simulink model "HvCoorn"  (R2022b)
settings: configuration reference "Icar05FusaMdlCfg" (kept outside this file)
undefined symbols (not defined in the file): BMSActSt_ACChrg, BMSActSt_DCChrg, BMSActSt_disconnect, BMSActSt_offline, BMSActSt_online, BMSActSt_undefined, BMSMainNegRlySt_Clsd_SC, BMSMainNegRlySt_Open_SC, BMSMainNegRlySt_StuckInClsd_SC, BMSMainNegRlySt_StuckInOpen_SC, BMSMainPosRlySt_Clsd_SC, BMSMainPosRlySt_Open_SC, BMSMainPosRlySt_StuckInClsd_SC, BMSPrecRlySt_StuckInOpen_SC, BMSReqSt_ACChrg, BMSReqSt_DCChrg, BMSReqSt_emergencyOffline, BMSReqSt_offline, BMSReqSt_online, Chrg_stCycleBookMod_SC, Chrg_stSingleBookMod_SC, CmpgMod_stInactv_SC, DCDCActSt_buck, DCDCActSt_connected, DCDCActSt_disconnected, DCDCReqSt_buck, DCDCReqSt_standby, EngStrtStop_RefuModDft_SC, EPBActSt_Appld_SC, GearLvr_stDrvGearD_SC, GearLvr_stDrvGearN_SC, GearLvr_stDrvGearP_SC, GearLvr_stDrvGearR_SC, hpp_bACChargeLinkIni_C, hpp_bACChargeLinkOKIni_C, hpp_bAcChgEnaIni_C, hpp_bAcChgPauseIni_C, hpp_bAcLinkTempErrIni_C, hpp_bBattWarmReqIni_C, hpp_bHvilHwErrIni_C, hpp_bHvilStOkIni_C, hpp_bHvRelayClsActIni_C, hpp_bHvRelayOpnActIni_C, hpp_bHvRelayStuckIni_C, hpp_bParked4ChDchgIni_C, hpp_bRemLvBatMntnReqIni_C, hpp_bStartUpReqIni_C, hpp_stHvilCanIni_C, hpp_stWarmTimeCfgRespIni_C, HvCoorn_bAuthEnaSwt_C, HvCoorn_bAuthFailSpdLimOvrd_C, HvCoorn_bAuthFailSpdLimOvrdVal_C, HvCoorn_bAuthStrt_C, HvCoorn_bBMSUnexpdDcnctFailEna_C, HvCoorn_bBuck2RdyBypDCDCEna_C, HvCoorn_bDCChrgFctCfg_C, HvCoorn_bDcChrgWkupEnaChrgLink_C, HvCoorn_bDCDcnct4ACEna_C, HvCoorn_bDCNotBuck2ShtdwnEna_C, HvCoorn_bDrvrLevNotRdyEna_C ... (+295)
libraries: ITKLib x213, simulink x61
(part 11 of 12)

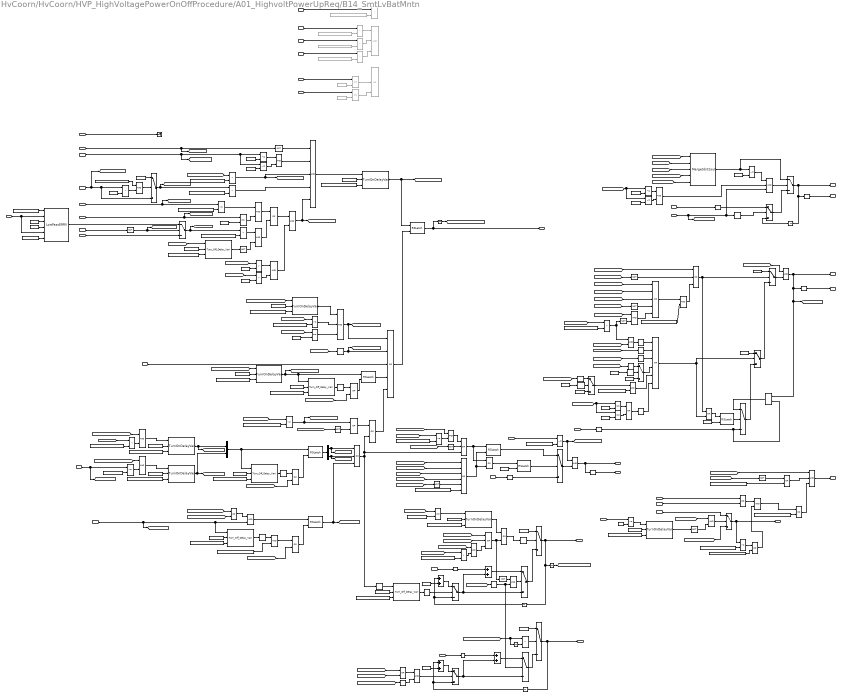
== system HvCoorn/HvCoorn/HVP_HighVoltagePowerOnOffProcedure/A01_HighvoltPowerUpReq/B14_SmtLvBatMntn ==
  icebs_pctLvBatSoh : Inport
  icbms_pctHVBatSOCDisp : Inport  Port=2
  icbms_tMaxBat : Inport  Port=3
  icbms_tMinBat : Inport  Port=4
  icebs_tLvBat : Inport  Port=5
  icebs_pctLvBatSoc : Inport  Port=6
  icebs_stSocPrcsn : Inport  Port=7
  icebs_uLvBat : Inport  Port=8
  idi_bKeyOn : Inport  Port=9
  ved_bInhbHvOn : Inport  Port=10
  icdc_stMode : Inport  Port=11
  icicm_bOTAOn : Inport  Port=12
  icicm_stHVReq : Inport  Port=13
  icicm_stOTAPwrMngtReq : Inport  Port=14
  HvCoorn_ctSmtBatMntnFailEER : Inport  Port=15
  iud_bEEIniFnsd : Inport  Port=16
  HvCoorn_stHVPOld : Inport  Port=17
  HvCoorn_ctSmtBatMntnSucsEER : Inport  Port=18
  ipf_bBD1CAN0x41CVld : Inport  Port=19
  idi_uPwrSply : Inport  Port=20
  ipf_bLIN9EBS0x34NodLostErr : Inport  Port=21
  HvCoorn_bSocWkupEER : Inport  Port=22
  HvCoorn_bTimerWkupReqEER : Inport  Port=23
  HvCoorn_stRemLvBatMntnFailRsnEER : Inport  Port=24
  idi_bEBSLinWkup : Inport  Port=25
  idi_bTimerWkup : Inport  Port=26
  HvCoorn_pctHVBatSocEER : Inport  Port=27
  idi_noBMSSocCounter : Inport  Port=28
  VehCfg_stLvBattTyp : Inport  Port=29
  AND : Logic  Inputs=5  OutDataTypeStr=boolean
  AND{1,6..7,9..10,12,17..20,22,24,26,29..30,32,36..40} (21 alike) : Logic  OutDataTypeStr=boolean
  AND{3,11,14,25,33..34} (6 alike) : Logic  Operator=OR  OutDataTypeStr=boolean
  AND13 : Logic  Operator=OR  Inputs=3  OutDataTypeStr=boolean
  AND15 : Logic  Operator=NOT  Inputs=3  OutDataTypeStr=boolean
  AND16 : Logic  Operator=NOT  Inputs=3  OutDataTypeStr=boolean
  AND2 : Logic  Commented=on  Inputs=3  OutDataTypeStr=boolean
  AND21 : Logic  Operator=OR  Inputs=6  OutDataTypeStr=boolean
  AND23 : Logic  Inputs=3  OutDataTypeStr=boolean
  AND27 : Logic  Operator=OR  Inputs=3  OutDataTypeStr=boolean
  AND28 : Logic  Operator=OR  Inputs=3  OutDataTypeStr=boolean
  AND31 : Logic  Operator=OR  Inputs=5  OutDataTypeStr=boolean
  AND35 : Logic  Inputs=3  OutDataTypeStr=boolean
  AND4 : Logic  Operator=OR  Inputs=5  OutDataTypeStr=boolean
  AND5 : Logic  Inputs=3  OutDataTypeStr=boolean
  AND8 : Logic  Commented=on  Operator=OR  Inputs=3  OutDataTypeStr=boolean
  Add{,1..3} (4 alike) : Sum  InputSameDT=on  SaturateOnIntegerOverflow=on
  Constant84 : Constant  Description=[1]  Value=LvBattTyp_stLiBatt_SC
      settings: AttributesFormatString=%<Description>
  CrCtl_tiFltVeh_C : Constant  Description=[0.02]  Value=HvCoorn_tiFiltLvVolt_C  SampleTime=-1
      settings: AttributesFormatString=%<Description>  CopyFcn=if exist('tl_reset_reviewflag','file')==2,tl_reset_reviewflag(gcbh);end  DeleteFcn=if exist('delete_tlblock','file')==2,delete_tlblock(gcbh);end  NameChangeFcn=if exist('rename_tlblock','file')==2,rename_tlblock(gcbh);end  OpenFcn=if exist('tl_open_blockdlg','file')==2,tl_open_blockdlg(gcbh);else,open_system(gcbh,'parameter');end
  Delay : Delay  DelayLength=1  InitialConditionSource=Input port
      settings: InputPortMap=u0,p4
  Delay1 : Delay  DelayLength=10  InitialCondition=0
  Delay2 : Delay  DelayLength=500  InitialCondition=0
  Demux : Demux  Outputs=2
  EdgeFalling{,1..3,5..6} (6 alike) : ITKLib/Memory/EdgeFalling  Tag=initial value = 0
      settings: SourceProductName=ITKC_Lib
  EdgeRising{,1..6,8,11..12} (10 alike) : ITKLib/Memory/EdgeRising  Tag=initial value = 0
      settings: SourceProductName=ITKC_Lib
  Equal : RelationalOperator  Commented=on  Operator===  OutDataTypeStr=boolean  RndMeth=Simplest  InputSameDT=off
  Equal1 : RelationalOperator  Commented=on  Operator===  OutDataTypeStr=boolean  RndMeth=Simplest  InputSameDT=off
  Equal2 : RelationalOperator  Operator=<  OutDataTypeStr=boolean
  Equal3 : RelationalOperator  Operator=~=  OutDataTypeStr=boolean
  Equal4 : RelationalOperator  Operator=~=  OutDataTypeStr=boolean
  Equal5 : RelationalOperator  OutDataTypeStr=boolean
  Equal7 : RelationalOperator  Operator=~=  OutDataTypeStr=boolean
  FALSE{1..4,6} (5 alike) : Constant  Description=FALSE  Value=0  OutDataTypeStr=boolean  SampleTime=-1
      settings: AttributesFormatString=%<Description>
  FALSE5 : Constant  Description=FALSE  Value=0  OutDataTypeStr=boolean
      settings: AttributesFormatString=%<Description>
  Greater : RelationalOperator  Commented=on  Operator=>  OutDataTypeStr=boolean
  Greater1 : RelationalOperator  Operator=<  OutDataTypeStr=boolean
  Greater{7,10..11,21} (4 alike) : RelationalOperator  Operator===  OutDataTypeStr=boolean
  Greater12 : RelationalOperator  Operator=<  OutDataTypeStr=boolean
  Greater{2,13..14,17..19} (6 alike) : RelationalOperator  Operator=>  OutDataTypeStr=boolean
  Greater{15..16,20,22} (4 alike) : RelationalOperator  Operator=~=  OutDataTypeStr=boolean
  Greater23 : RelationalOperator  Operator=<=  OutDataTypeStr=boolean
  Greater26 : RelationalOperator  Operator=<=  OutDataTypeStr=boolean
  Greater3 : RelationalOperator  Commented=on  Operator=>  OutDataTypeStr=boolean
  Greater4 : RelationalOperator  Commented=on  Operator=<  OutDataTypeStr=boolean
  Greater5 : RelationalOperator  Commented=on  Operator=>  OutDataTypeStr=boolean
  Greater6 : RelationalOperator  Operator=<=  OutDataTypeStr=boolean
  Greater8 : RelationalOperator  Operator=<  OutDataTypeStr=boolean
  Greater9 : RelationalOperator  OutDataTypeStr=boolean
  LowPassERRV1 : ITKLib/Filter/LowPassERRV
      settings: SourceProductName=ITKC_Lib
  Merge5bit2out : ITKLib/BitOperation/Merge5bit2out
      settings: SourceProductName=ITKC_Lib
  Mux : Mux  Inputs=2
  Not{,1..9} (10 alike) : Logic  Operator=NOT  AllPortsSameDT=off  OutDataTypeStr=boolean
  OR : Logic  Operator=OR  Inputs=3  OutDataTypeStr=boolean
  OR1 : Logic  OutDataTypeStr=boolean
  OR{2..5,7..8,10..13} (10 alike) : Logic  Operator=OR  OutDataTypeStr=boolean
  OR6 : Logic  Operator=OR  Inputs=6  OutDataTypeStr=boolean
  OR9 : Logic  OutDataTypeStr=boolean
  RSLatch{,1..6} (7 alike) : ITKLib/Memory/RSLatch
      settings: SourceProductName=ITKC_Lib
  Relational Operator1 : RelationalOperator  Operator===  OutDataTypeStr=boolean  InputSameDT=off
  Relational Operator5 : RelationalOperator  Operator=~=  OutDataTypeStr=boolean  InputSameDT=off
  Signal Copy{,1..7} (8 alike) : SignalConversion  OverrideOpt=off
  Switch{,1..9,11..17} (17 alike) : Switch  Criteria=u2 ~= 0  SaturateOnIntegerOverflow=off  InputSameDT=off
      settings: AttributesFormatString=Criteria : %<Criteria>
  TRUE : Constant  Description=TRUE  OutDataTypeStr=boolean  SampleTime=-1
      settings: AttributesFormatString=%<Description>
  TRUE1 : Constant  Description=TRUE  OutDataTypeStr=boolean  SampleTime=-1
      settings: AttributesFormatString=%<Description>
  TRUE2 : Constant  Description=TRUE  OutDataTypeStr=boolean
      settings: AttributesFormatString=%<Description>
  TRUE3 : Constant  Description=TRUE  OutDataTypeStr=boolean  SampleTime=-1
      settings: AttributesFormatString=%<Description>
  TaskTime_s{1..13} (13 alike) : Constant  Value=TaskTime_10ms
      settings: AttributesFormatString=[0.01]
  Terminator : Terminator
  TurnOnDelayVari{,1..6} (7 alike) : ITKLib/TimeCounter/TurnOnDelayVari
      settings: AttributesFormatString=TurnOnDelay  SourceProductName=ITKC_Lib
  Turn_Off_Delay_Vari{,1..4} (5 alike) : ITKLib/TimeCounter/Turn_Off_Delay_Vari
      settings: AttributesFormatString=TurnOffDelay  SourceProductName=ITKC_Lib
  Unit Delay : UnitDelay  SampleTime=-1  HasFrameUpgradeWarning=on
      settings: AttributesFormatString=<initial=%<x0>>
  Unit Delay1 : UnitDelay  SampleTime=-1  HasFrameUpgradeWarning=on
      settings: AttributesFormatString=<initial=%<x0>>
  Unit Delay2 : UnitDelay  SampleTime=-1  HasFrameUpgradeWarning=on
      settings: AttributesFormatString=<initial=%<x0>>
  UnitDelay : UnitDelay  SampleTime=-1  HasFrameUpgradeWarning=on
      settings: AttributesFormatString=<Initial=%<x0>>
  UnitDelay1 : UnitDelay  SampleTime=-1  HasFrameUpgradeWarning=on
      settings: AttributesFormatString=<Initial=%<x0>>
  UnitDelay2 : UnitDelay  SampleTime=-1  HasFrameUpgradeWarning=on
      settings: AttributesFormatString=<Initial=%<x0>>
  hpp_tiRemHvBatPrecdngSet_C : Constant  Description=[75]  Commented=on  Value=HvCoorn_pctLvBatSohRemMntnThd_C
      settings: AttributesFormatString=%<Description>
  hpp_tiRemHvBatPrecdngSet_C1 : Constant  Description=[3]  Value=HvCoorn_ctSmtBatMntnFailThd_C
      settings: AttributesFormatString=%<Description>
  hpp_tiRemHvBatPrecdngSet_C10 : Constant  Description=[70]  Value=HvCoorn_pctHvBatSocMntnFailClr_C
      settings: AttributesFormatString=%<Description>
  hpp_tiRemHvBatPrecdngSet_C11 : Constant  Description=[5400]  Value=HvCoorn_tiRemMntnActvOverThd_C
      settings: AttributesFormatString=%<Description>
  hpp_tiRemHvBatPrecdngSet_C12 : Constant  Description=[15]  Value=HvCoorn_tiRemMntnDcdcNoBuckEx_C
      settings: AttributesFormatString=%<Description>
  hpp_tiRemHvBatPrecdngSet_C13 : Constant  Description=[13]  Value=HvCoorn_uLvBatRemMntnExThd_C
      settings: AttributesFormatString=%<Description>
  hpp_tiRemHvBatPrecdngSet_C14 : Constant  Description=[15]  Value=HvCoorn_tiRemMntnLvVoltExThd_C
      settings: AttributesFormatString=%<Description>
  hpp_tiRemHvBatPrecdngSet_C15 : Constant  Description=[70]  Value=HvCoorn_pctHvBatSocMntnFailClr_C
      settings: AttributesFormatString=%<Description>
  hpp_tiRemHvBatPrecdngSet_C16 : Constant  Description=[70]  Value=HvCoorn_pctHvBatSocMntnFailClr_C
      settings: AttributesFormatString=%<Description>
  hpp_tiRemHvBatPrecdngSet_C17 : Constant  Description=[180]  Value=HvCoorn_tiMntnKeyOffThd_C
      settings: AttributesFormatString=%<Description>
  hpp_tiRemHvBatPrecdngSet_C18 : Constant  Description=[8]  Value=HvCoorn_pctHvBatSocRemMntnExThd_C
      settings: AttributesFormatString=%<Description>
  hpp_tiRemHvBatPrecdngSet_C19 : Constant  Description=[1800]  Value=HvCoorn_tiRemMntnOverKeepRst_C
      settings: AttributesFormatString=%<Description>
  hpp_tiRemHvBatPrecdngSet_C2 : Constant  Description=[8]  Value=HvCoorn_pctHvBatSocRemMntnThd_C
      settings: AttributesFormatString=%<Description>
  hpp_tiRemHvBatPrecdngSet_C20 : Constant  Description=[1800]  Value=HvCoorn_tiRemMntnFailKeepRst_C
      settings: AttributesFormatString=%<Description>
  hpp_tiRemHvBatPrecdngSet_C21 : Constant  Description=[1]  Value=HvCoorn_tiRemMntnFailCtDly_C
      settings: AttributesFormatString=%<Description>
  hpp_tiRemHvBatPrecdngSet_C22 : Constant  Description=[1800]  Value=HvCoorn_tiRemMntnFltKeepRst_C
      settings: AttributesFormatString=%<Description>
  hpp_tiRemHvBatPrecdngSet_C23 : Constant  Description=[0]  Value=HvCoorn_bRemMntnFailKeepRstEna_C
      settings: AttributesFormatString=%<Description>
  hpp_tiRemHvBatPrecdngSet_C24 : Constant  Description=[1]  Value=HvCoorn_bSmtBatSocZeroOvrdEna_C
      settings: AttributesFormatString=%<Description>
  hpp_tiRemHvBatPrecdngSet_C25 : Constant  Description=[0]  Value=HvCoorn_bVehNetWkupInhbHvOnByp_C
      settings: AttributesFormatString=%<Description>
  hpp_tiRemHvBatPrecdngSet_C26 : Constant  Description=[0]  Value=HvCoorn_bTimerWkupReqShd_C
      settings: AttributesFormatString=%<Description>
  hpp_tiRemHvBatPrecdngSet_C27 : Constant  Description=[1]  Value=HvCoorn_bSocWkupInactvEna_C
      settings: AttributesFormatString=%<Description>
  hpp_tiRemHvBatPrecdngSet_C28 : Constant  Description=[25]  Value=HvCoorn_tiRemMntnDCBuckRst_C
      settings: AttributesFormatString=%<Description>
  hpp_tiRemHvBatPrecdngSet_C29 : Constant  Description=[0.1]  Value=HvCoorn_tiLvBatMntnReqThd_C
      settings: AttributesFormatString=%<Description>
  hpp_tiRemHvBatPrecdngSet_C3 : Constant  Description=[-20]  Commented=on  Value=HvCoorn_tMaxBatRemMntnThd_C
      settings: AttributesFormatString=%<Description>
  hpp_tiRemHvBatPrecdngSet_C30 : Constant  Description=[1]  Value=HvCoorn_bSocWkupEna_C
      settings: AttributesFormatString=%<Description>
  hpp_tiRemHvBatPrecdngSet_C31 : Constant  Description=[1]  Value=HvCoorn_bVehNetWkupJudgByp_C
      settings: AttributesFormatString=%<Description>
  hpp_tiRemHvBatPrecdngSet_C32 : Constant  Description=[8]  Value=HvCoorn_pctHvBatSocNetWkupThd_C
      settings: AttributesFormatString=%<Description>
  hpp_tiRemHvBatPrecdngSet_C33 : Constant  Description=[0.01]  Value=HvCoorn_tiBMSSocCounterThd_C
      settings: AttributesFormatString=%<Description>
  hpp_tiRemHvBatPrecdngSet_C34 : Constant  Description=[1]  Value=HvCoorn_bVehNetWkupSocByp_C
      settings: AttributesFormatString=%<Description>
  hpp_tiRemHvBatPrecdngSet_C4 : Constant  Description=[-20]  Commented=on  Value=HvCoorn_tMinBatRemMntnThd_C
      settings: AttributesFormatString=%<Description>
  hpp_tiRemHvBatPrecdngSet_C5 : Constant  Description=[-30]  Commented=on  Value=HvCoorn_tLvBatRemMntnThd_C
      settings: AttributesFormatString=%<Description>
  hpp_tiRemHvBatPrecdngSet_C6 : Constant  Description=[70]  Value=HvCoorn_pctLvBatSocRemMntnThd_C
      settings: AttributesFormatString=%<Description>
  hpp_tiRemHvBatPrecdngSet_C7 : Constant  Description=[11.8]  Value=HvCoorn_uLvBatRemMntnThd_C
      settings: AttributesFormatString=%<Description>
  hpp_tiRemHvBatPrecdngSet_C8 : Constant  Description=[1200]  Value=HvCoorn_tiRemMntnSocMaxExThd_C
      settings: AttributesFormatString=%<Description>
  hpp_tiRemHvBatPrecdngSet_C9 : Constant  Description=[90]  Value=HvCoorn_pctLvBatSocRemMntnEx_C
      settings: AttributesFormatString=%<Description>
  icdc_disconnected : Constant  Description=[1]  Value=DCDCActSt_buck
      settings: AttributesFormatString=[1]
  icdc_disconnected1 : Constant  Description=[1]  Value=DCDCActSt_buck
      settings: AttributesFormatString=[1]
  single : Constant  Value=0.1  OutDataTypeStr=single  SampleTime=-1
      settings: AttributesFormatString=%<OutDataTypeStr>
  single1 : Constant  Value=0.1  OutDataTypeStr=single  SampleTime=-1
      settings: AttributesFormatString=%<OutDataTypeStr>
  single2 : Constant  Value=0.01  OutDataTypeStr=single  SampleTime=-1
      settings: AttributesFormatString=%<OutDataTypeStr>
  single3 : Constant  Value=100  OutDataTypeStr=single  SampleTime=-1
      settings: AttributesFormatString=%<OutDataTypeStr>
  uint1 : Constant  Value=2  OutDataTypeStr=uint8  SampleTime=-1
      settings: AttributesFormatString=%<OutDataTypeStr>
  uint10 : Constant  Value=0  OutDataTypeStr=uint16  SampleTime=-1
      settings: AttributesFormatString=%<OutDataTypeStr>
  uint11 : Constant  Value=90  OutDataTypeStr=uint8  SampleTime=-1
      settings: AttributesFormatString=%<OutDataTypeStr>
  uint12 : Constant  Value=89  OutDataTypeStr=uint8  SampleTime=-1
      settings: AttributesFormatString=%<OutDataTypeStr>
  uint13 : Constant  Value=90  OutDataTypeStr=uint8  SampleTime=-1
      settings: AttributesFormatString=%<OutDataTypeStr>
  uint14 : Constant  Value=89  OutDataTypeStr=uint8  SampleTime=-1
      settings: AttributesFormatString=%<OutDataTypeStr>
  uint15 : Constant  Value=0  OutDataTypeStr=uint8  SampleTime=-1
      settings: AttributesFormatString=%<OutDataTypeStr>
  uint16 : Constant  OutDataTypeStr=uint16  SampleTime=-1
      settings: AttributesFormatString=%<OutDataTypeStr>
  uint2 : Constant  Commented=on  Value=2  OutDataTypeStr=uint8  SampleTime=-1
      settings: AttributesFormatString=%<OutDataTypeStr>
  uint3 : Constant  Commented=on  OutDataTypeStr=uint8  SampleTime=-1
      settings: AttributesFormatString=%<OutDataTypeStr>
  uint4 : Constant  Value=0  OutDataTypeStr=uint8  SampleTime=-1
      settings: AttributesFormatString=%<OutDataTypeStr>
  uint5 : Constant  OutDataTypeStr=uint8  SampleTime=-1
      settings: AttributesFormatString=%<OutDataTypeStr>
  uint6 : Constant  Value=89  OutDataTypeStr=uint8  SampleTime=-1
      settings: AttributesFormatString=%<OutDataTypeStr>
  uint7 : Constant  Value=90  OutDataTypeStr=uint8  SampleTime=-1
      settings: AttributesFormatString=%<OutDataTypeStr>
  uint8 : Constant  Value=2  OutDataTypeStr=uint8  SampleTime=-1
      settings: AttributesFormatString=%<OutDataTypeStr>
  uint9 : Constant  Value=0  OutDataTypeStr=uint8  SampleTime=-1
      settings: AttributesFormatString=%<OutDataTypeStr>
  HvCoorn_bLvBatMntnReq : Outport  VectorParamsAs1DForOutWhenUnconnected=off
  HvCoorn_bSocWkup : Outport  Port=2  VectorParamsAs1DForOutWhenUnconnected=off
  HvCoorn_ctSmtBatMntnFailEEW : Outport  Port=3  VectorParamsAs1DForOutWhenUnconnected=off
  HvCoorn_stRemLvBatMntnFailRsn : Outport  Port=4  VectorParamsAs1DForOutWhenUnconnected=off
  HvCoorn_bTimerWkupReq : Outport  Port=5  VectorParamsAs1DForOutWhenUnconnected=off
  HvCoorn_ctSmtBatMntnSucsEEW : Outport  Port=6  VectorParamsAs1DForOutWhenUnconnected=off
  HvCoorn_bVehNetWkupEna : Outport  Port=7  VectorParamsAs1DForOutWhenUnconnected=off
  HvCoorn_bSocWkupEEW : Outport  Port=8  VectorParamsAs1DForOutWhenUnconnected=off
  HvCoorn_bTimerWkupReqEEW : Outport  Port=9  VectorParamsAs1DForOutWhenUnconnected=off
  HvCoorn_stRemLvBatMntnFailRsnEEW : Outport  Port=10  VectorParamsAs1DForOutWhenUnconnected=off
  HvCoorn_pctHVBatSocEEW : Outport  Port=11  VectorParamsAs1DForOutWhenUnconnected=off
  wires:
  icebs_pctLvBatSoh/1 -> Greater/1
  hpp_tiRemHvBatPrecdngSet_C/1 -> Greater/2
  hpp_tiRemHvBatPrecdngSet_C1/1 -> Greater1/2
  [HvCoorn_ctSmtBatMntnFailEEW] -> Greater1/1
  Switch9/1 -> [HvCoorn_pctHVBatSOCDisp], Greater2/1
  hpp_tiRemHvBatPrecdngSet_C2/1 -> Greater2/2
  hpp_tiRemHvBatPrecdngSet_C3/1 -> Greater3/2
  icbms_tMaxBat/1 -> Greater3/1
  icbms_tMinBat/1 -> Greater4/1
  hpp_tiRemHvBatPrecdngSet_C4/1 -> Greater4/2
  hpp_tiRemHvBatPrecdngSet_C5/1 -> Greater5/2
  icebs_tLvBat/1 -> Greater5/1
  hpp_tiRemHvBatPrecdngSet_C6/1 -> Greater6/2
  icebs_pctLvBatSoc/1 -> Greater6/1, [icebs_pctLvBatSoc]
  Greater6/1 -> AND1/1
  Greater3/1 -> AND2/1
  Greater4/1 -> AND2/2
  Greater5/1 -> AND2/3
  AND1/1 -> AND3/1
  icebs_stSocPrcsn/1 -> Greater7/1, [icebs_stSocPrcsn]
  uint8/1 -> Greater7/2  "lowr10"
  Greater7/1 -> AND1/2
  Switch8/1 -> [icebs_uLvBat], Greater8/1
  hpp_tiRemHvBatPrecdngSet_C7/1 -> Greater8/2
  TurnOnDelayVari5/1 -> RSLatch/1, [HvCoorn_bLvBatMntnReqSet]  "HvCoorn_bLvBatMntnReqSet"
  RSLatch/1 -> UnitDelay/1, HvCoorn_bLvBatMntnReq/1  "HvCoorn_bLvBatMntnReq"
  UnitDelay/1 -> [HvCoorn_bRemLvBatMntnReqOld]
  [HvCoorn_bRemLvBatMntnReqOld] -> TurnOnDelayVari/1
  hpp_tiRemHvBatPrecdngSet_C8/1 -> TurnOnDelayVari/3
  TaskTime_s2/1 -> TurnOnDelayVari/2
  [icebs_pctLvBatSoc] -> Greater9/1
  hpp_tiRemHvBatPrecdngSet_C9/1 -> Greater9/2
  uint1/1 -> Greater10/2  "lowr10"
  [icebs_stSocPrcsn] -> Greater10/1
  Greater9/1 -> AND5/2
  TurnOnDelayVari/1 -> AND5/1
  Greater10/1 -> AND5/3
  AND5/1 -> AND4/1, [HvCoorn_bMntnEx1]
  EdgeRising/1 -> [HvCoorn_bMntnEx2], AND4/2
  TaskTime_s1/1 -> TurnOnDelayVari1/2
  hpp_tiRemHvBatPrecdngSet_C11/1 -> TurnOnDelayVari1/3
  [HvCoorn_bRemLvBatMntnReqOld] -> TurnOnDelayVari1/1
  [HvCoorn_bRemLvBatMntnReqOld] -> AND6/1
  hpp_tiRemHvBatPrecdngSet_C12/1 -> TurnOnDelayVari2/3
  TaskTime_s3/1 -> TurnOnDelayVari2/2
  icdc_stMode/1 -> [icdc_stMode], Relational Operator5/1
  icdc_disconnected/1 -> Relational Operator5/2
  Relational Operator5/1 -> AND6/2
  hpp_tiRemHvBatPrecdngSet_C13/1 -> Greater12/2
  [icebs_uLvBat] -> Greater12/1
  TaskTime_s4/1 -> TurnOnDelayVari3/2
  hpp_tiRemHvBatPrecdngSet_C14/1 -> TurnOnDelayVari3/3
  [HvCoorn_bRemLvBatMntnReqOld] -> AND7/1
  Greater12/1 -> AND7/2
  AND7/1 -> TurnOnDelayVari3/1
  AND4/1 -> RSLatch/2  "HvCoorn_bRemLvBatMntnEx"
  icicm_stHVReq/1 -> Equal/1
  uint2/1 -> Equal1/2
  uint3/1 -> Equal/2
  Equal/1 -> AND8/2
  Equal1/1 -> AND8/3
  icicm_stOTAPwrMngtReq/1 -> Equal1/1
  ved_bInhbHvOn/1 -> [ved_bInhbHvOn], AND12/2, Turn_Off_Delay_Vari4/1
  TurnOnDelayVari2/1 -> Mux/2, [HvCoorn_bMntnEx7]
  TurnOnDelayVari3/1 -> Mux/1, [HvCoorn_bMntnEx5]
  AND11/1 -> AND4/5
  AND28/1 -> EdgeRising2/1, AND11/2, AND13/3  "HvCoorn_bRemLvBatMntnFail"
  [iud_bEEIniFnsd] -> EdgeRising1/1
  EdgeFalling6/1 -> Switch1/2
  Switch1/1 -> Add/2, Switch/3
  uint5/1 -> Add1/2
  Unit Delay/1 -> Add1/1, Switch1/3
  Add1/1 -> Switch1/1
  Add/1 -> Switch/1
  HvCoorn_ctSmtBatMntnFailEER/1 -> Signal Copy/1
  Switch/1 -> Switch2/3
  uint4/1 -> Switch2/1
  idi_bKeyOn/1 -> [idi_bKeyOn], AND15/1
  AND15/1 -> AND/1
  OR1/1 -> Switch/2
  OR/1 -> AND16/1, OR3/2
  AND16/1 -> OR1/1
  [idi_bKeyOn] -> EdgeRising/1
  Signal Copy/1 -> Add/1  "HvCoorn_ctSmtBatMntnFailEER"
  Switch2/1 -> UnitDelay1/1, Unit Delay/1, HvCoorn_ctSmtBatMntnFailEEW/1
  AND3/1 -> AND17/1
  single/1 -> Greater13/2
  [icebs_pctLvBatSoc] -> Greater13/1
  [icebs_uLvBat] -> Greater14/1
  single1/1 -> Greater14/2
  Greater13/1 -> AND18/1
  Greater14/1 -> AND18/2
  AND18/1 -> AND17/2
  AND17/1 -> [HvCoorn_bEbsSocEna], AND/5
  HvCoorn_stHVPOld/1 -> [HvCoorn_stHVPOld], Greater15/1, Greater16/1
  uint6/1 -> Greater15/2
  uint7/1 -> Greater16/2
  Greater15/1 -> AND19/1
  Greater16/1 -> AND19/2
  AND19/1 -> AND/2
  [HvCoorn_bMntnEx1] -> OR/1
  [HvCoorn_bMntnEx2] -> OR/2
  EdgeRising3/1 -> Switch2/2
  [HvCoorn_bMntnEx4] -> AND9/1
  AND9/1 -> OR/3
  hpp_tiRemHvBatPrecdngSet_C15/1 -> Greater17/2
  [icebs_pctLvBatSoc] -> Greater17/1
  Greater17/1 -> AND9/2
  Greater18/1 -> Not3/1, AND20/1
  [icebs_pctLvBatSoc] -> Greater18/1
  hpp_tiRemHvBatPrecdngSet_C16/1 -> Greater18/2
  [HvCoorn_bMntnEx4] -> AND20/2
  uint10/1 -> Switch3/1
  [HvCoorn_ctSmtBatMntnFailEEW] -> UnitDelay2/1, Greater19/1
  Greater19/1 -> Switch3/2
  UnitDelay2/1 -> Greater19/2
  Switch4/1 -> Switch3/3
  Signal Copy1/1 -> Add2/1  "HvCoorn_ctSmtBatMntnSucsEER"
  HvCoorn_ctSmtBatMntnSucsEER/1 -> Signal Copy1/1
  Add2/1 -> Switch4/1
  EdgeRising1/1 -> OR1/2, Switch4/2
  Switch3/1 -> Unit Delay1/1, HvCoorn_ctSmtBatMntnSucsEEW/1
  Add3/1 -> Switch5/1
  Unit Delay1/1 -> Switch5/3, Add3/1
  uint16/1 -> Add3/2
  Switch5/1 -> Add2/2, Switch4/3
  [HvCoorn_bMntnEx2] -> OR2/2
  [HvCoorn_bMntnEx1] -> OR2/1
  OR2/1 -> AND22/1
  AND22/1 -> Switch5/2
  EdgeFalling/1 -> AND22/2
  [HvCoorn_bRemLvBatMntnReqOld] -> EdgeFalling/1
  UnitDelay1/1 -> [HvCoorn_ctSmtBatMntnFailEEW]
  Greater1/1 -> [HvCoorn_bMntnEna], AND/3
  Greater2/1 -> AND/4
  AND20/1 -> EdgeRising4/1
  OR3/1 -> EdgeRising3/1
  AND6/1 -> TurnOnDelayVari2/1
  [idi_bKeyOn] -> Turn_Off_Delay_Vari/1
  TaskTime_s5/1 -> Turn_Off_Delay_Vari/2
  hpp_tiRemHvBatPrecdngSet_C17/1 -> Turn_Off_Delay_Vari/3
  Greater8/1 -> AND24/1
  Turn_Off_Delay_Vari/1 -> Not/1
  Not/1 -> AND24/2
  AND24/1 -> AND3/2
  AND25/1 -> AND11/1
  Greater26/1 -> [HvCoorn_bHVBatSocLow], AND25/1
  Not2/1 -> AND25/2
  [HvCoorn_bMntnEna] -> Not2/1
  TRUE/1 -> Switch7/1
  FALSE1/1 -> Switch6/1
  AND39/1 -> HvCoorn_bSocWkup/1, Delay/1, [HvCoorn_bSocWkup], Signal Copy2/1
  Not3/1 -> AND26/2
  [HvCoorn_bMntnEx4] -> AND26/1
  [HvCoorn_bMntnEna] -> Not5/1
  [HvCoorn_bMntnEx1] -> EdgeRising6/1
  [HvCoorn_bMntnEx2] -> EdgeRising8/1
  AND26/1 -> AND31/5
  AND27/1 -> Switch6/2, OR7/1
  Switch7/1 -> Switch6/3
  [HvCoorn_bHVBatSocLow] -> AND27/1
  Not5/1 -> AND27/2
  [HvCoorn_bMntnEx5] -> AND31/1
  [HvCoorn_bMntnEx6] -> AND31/2
  [HvCoorn_bMntnEx7] -> AND31/3
  [HvCoorn_stHVPOld] -> Greater11/1, Greater21/1
  uint12/1 -> Greater11/2
  Greater21/1 -> OR8/2
  Greater11/1 -> OR8/1
  uint11/1 -> Greater21/2
  OR8/1 -> EdgeRising12/1
  hpp_tiRemHvBatPrecdngSet_C10/1 -> Greater23/2
  [icebs_pctLvBatSoc] -> Greater23/1
  [HvCoorn_bMntnEx4] -> AND10/1
  Greater23/1 -> AND10/2
  [HvCoorn_bMntnEx1] -> AND21/1
  [HvCoorn_bMntnEx2] -> AND21/2
  AND21/1 -> RSLatch1/2, OR5/2
  [HvCoorn_bSocWkup] -> AND21/3
  Not1/1 -> [ipf_bBD1CAN0x41CVld], Switch8/2
  idi_uPwrSply/1 -> Switch8/3
  Not6/1 -> AND31/4
  [ipf_bBD1CAN0x41CVld] -> Not6/1
  [ipf_bBD1CAN0x41CVld] -> EdgeRising11/1
  [ipf_bBD1CAN0x41CVld] -> Not7/1
  Not7/1 -> AND13/2
  OR6/1 -> OR7/2, Switch7/2
  AND10/1 -> AND13/1
  [HvCoorn_bEbsSocEna] -> AND23/1
  AND23/1 -> HvCoorn_bVehNetWkupEna/1
  hpp_tiRemHvBatPrecdngSet_C18/1 -> Greater26/2
  [HvCoorn_pctHVBatSOCDisp] -> Greater26/1
  EdgeRising4/1 -> OR6/1
  EdgeRising6/1 -> OR6/2
  EdgeRising8/1 -> OR6/3
  RSLatch3/1 -> AND4/4
  [icdc_stMode] -> Relational Operator1/1
  icdc_disconnected1/1 -> Relational Operator1/2
  ipf_bBD1CAN0x41CVld/1 -> Terminator/1
  ipf_bLIN9EBS0x34NodLostErr/1 -> Not1/1
  [HvCoorn_bMntnEna] -> Not4/1
  Not4/1 -> AND21/5
  [HvCoorn_bHVBatSocLow] -> AND21/4
  TurnOnDelayVari1/1 -> [HvCoorn_bMntnEx4], Turn_Off_Delay_Vari1/1, RSLatch3/1
  Turn_Off_Delay_Vari1/1 -> EdgeFalling3/1
  TaskTime_s6/1 -> Turn_Off_Delay_Vari1/2
  hpp_tiRemHvBatPrecdngSet_C19/1 -> Turn_Off_Delay_Vari1/3
  hpp_tiRemHvBatPrecdngSet_C20/1 -> Turn_Off_Delay_Vari2/3
  TaskTime_s7/1 -> Turn_Off_Delay_Vari2/2
  Turn_Off_Delay_Vari2/1 -> EdgeFalling5/1
  Mux/1 -> Turn_Off_Delay_Vari2/1, RSLatch2/1
  TaskTime_s8/1 -> Turn_Off_Delay_Vari3/2
  hpp_tiRemHvBatPrecdngSet_C21/1 -> Turn_Off_Delay_Vari3/3
  EdgeRising2/1 -> Turn_Off_Delay_Vari3/1
  Turn_Off_Delay_Vari3/1 -> EdgeFalling6/1
  AND12/1 -> RSLatch4/1
  RSLatch4/1 -> AND28/3, [HvCoorn_bMntnEx6]
  [HvCoorn_bRemLvBatMntnReqOld] -> OR4/2
  [HvCoorn_bLvBatMntnReqSet] -> OR4/1
  OR4/1 -> AND12/1
  Turn_Off_Delay_Vari4/1 -> EdgeFalling2/1
  TaskTime_s9/1 -> Turn_Off_Delay_Vari4/2
  hpp_tiRemHvBatPrecdngSet_C22/1 -> Turn_Off_Delay_Vari4/3
  EdgeFalling2/1 -> AND29/1
  hpp_tiRemHvBatPrecdngSet_C23/1 -> AND29/2
  icbms_pctHVBatSOCDisp/1 -> [icbms_pctHVBatSOCDisp], Equal2/1, Switch9/3
  single2/1 -> Equal2/2
  single3/1 -> Switch9/1
  Equal2/1 -> AND30/2
  AND30/1 -> Switch9/2
  hpp_tiRemHvBatPrecdngSet_C24/1 -> AND30/1
  [ved_bInhbHvOn] -> Not8/1
  hpp_tiRemHvBatPrecdngSet_C25/1 -> OR13/2
  hpp_tiRemHvBatPrecdngSet_C26/1 -> AND21/6
  AND13/1 -> OR5/1, RSLatch1/1
  AND31/1 -> AND32/1
  AND32/1 -> AND27/3
  hpp_tiRemHvBatPrecdngSet_C27/1 -> AND32/2
  RSLatch2/1 -> Demux/1
  Demux/2 -> [HvCoorn_bFail3], AND28/2
  Demux/1 -> [HvCoorn_bFail2], AND28/1
  TaskTime_s10/1 -> TurnOnDelayVari4/2
  hpp_tiRemHvBatPrecdngSet_C28/1 -> TurnOnDelayVari4/3
  Relational Operator1/1 -> TurnOnDelayVari4/1
  TurnOnDelayVari4/1 -> OR3/1
  EdgeFalling3/1 -> AND14/1
  AND14/1 -> RSLatch3/2
  [HvCoorn_bMntnEx2] -> AND14/2
  [HvCoorn_bMntnEx2] -> AND33/2
  EdgeFalling5/1 -> AND33/1
  AND33/1 -> RSLatch2/2
  [HvCoorn_bMntnEx2] -> AND34/2
  AND29/1 -> AND34/1
  AND34/1 -> RSLatch4/2
  Switch11/1 -> Switch7/3
  Delay/1 -> Switch11/1
  Signal Copy2/1 -> HvCoorn_bSocWkupEEW/1
  HvCoorn_bSocWkupEER/1 -> Signal Copy3/1
  Signal Copy3/1 -> Switch11/3, Delay/2  "HvCoorn_bSocWkupEER"
  FALSE3/1 -> RSLatch5/2
  RSLatch5/1 -> Switch12/2  "HvCoorn_bTimerWkupKeep"
  RSLatch1/1 -> Switch12/1
  AND38/1 -> Signal Copy5/1, HvCoorn_bTimerWkupReq/1
  OR5/1 -> RSLatch5/1
  HvCoorn_bTimerWkupReqEER/1 -> Signal Copy4/1
  Signal Copy4/1 -> Switch12/3  "HvCoorn_bTimerWkupReqEER"
  Signal Copy5/1 -> HvCoorn_bTimerWkupReqEEW/1
  FALSE4/1 -> RSLatch6/2
  OR7/1 -> RSLatch6/1
  RSLatch6/1 -> Switch11/2
  EdgeRising11/1 -> Switch13/1
  Switch13/1 -> OR6/4
  Delay1/1 -> Switch13/2
  FALSE2/1 -> Switch13/3
  TRUE1/1 -> Delay1/1
  FALSE5/1 -> LowPassERRV1/4
  TaskTime_s11/1 -> LowPassERRV1/6
  TRUE2/1 -> LowPassERRV1/3
  icebs_uLvBat/1 -> LowPassERRV1/5, LowPassERRV1/2
  CrCtl_tiFltVeh_C/1 -> LowPassERRV1/1
  LowPassERRV1/1 -> Switch8/1  "HvCoorn_uLvBat"
  icicm_bOTAOn/1 -> AND4/3
  TaskTime_s12/1 -> TurnOnDelayVari5/2
  hpp_tiRemHvBatPrecdngSet_C29/1 -> TurnOnDelayVari5/3
  AND/1 -> TurnOnDelayVari5/1  "HvCoorn_bLvBatMntnReqSetRaw"
  VehCfg_stLvBattTyp/1 -> Equal3/1
  Constant84/1 -> Equal3/2
  Equal3/1 -> AND38/1, [HvCoorn_bNotLiBattCfg]
  Switch12/1 -> AND38/2
  [HvCoorn_bNotLiBattCfg] -> AND39/1
  Switch6/1 -> AND39/2
  Merge5bit2out/1 -> Switch14/1, Equal4/1
  uint9/1 -> Equal4/2
  Switch14/1 -> Unit Delay2/1, Signal Copy6/1, HvCoorn_stRemLvBatMntnFailRsn/1
  Switch15/1 -> Switch14/3
  Unit Delay2/1 -> Switch15/3
  Signal Copy6/1 -> HvCoorn_stRemLvBatMntnFailRsnEEW/1
  HvCoorn_stRemLvBatMntnFailRsnEER/1 -> Signal Copy7/1
  Signal Copy7/1 -> Switch15/1  "HvCoorn_stRemLvBatMntnFailRsnEER"
  Equal4/1 -> AND35/1
  AND35/1 -> Switch14/2
  iud_bEEIniFnsd/1 -> AND35/3, EdgeRising5/1, [iud_bEEIniFnsd]
  EdgeRising5/1 -> Switch15/2
  EdgeRising12/1 -> OR6/6
  TRUE3/1 -> Delay2/1
  FALSE6/1 -> Switch16/3
  Delay2/1 -> Switch16/2
  [HvCoorn_bHVBatSocLow] -> EdgeFalling1/1
  EdgeFalling1/1 -> Switch16/1
  Switch16/1 -> AND36/1
  AND36/1 -> OR6/5
  hpp_tiRemHvBatPrecdngSet_C30/1 -> AND36/2
  uint13/1 -> Greater22/2
  [HvCoorn_stHVPOld] -> Greater20/1, Greater22/1
  uint14/1 -> Greater20/2
  Greater22/1 -> OR9/2
  Greater20/1 -> OR9/1
  [HvCoorn_bMntnEx6] -> Merge5bit2out/1
  OR9/1 -> AND35/2
  [HvCoorn_bFail2] -> Merge5bit2out/2
  [HvCoorn_bFail3] -> Merge5bit2out/3
  [HvCoorn_bHVBatSocLow] -> Merge5bit2out/4
  [ved_bInhbHvOn] -> Merge5bit2out/5
  OR10/1 -> AND23/3
  hpp_tiRemHvBatPrecdngSet_C31/1 -> OR10/2
  idi_bEBSLinWkup/1 -> OR11/1
  idi_bTimerWkup/1 -> OR11/2
  OR11/1 -> AND37/1
  AND37/1 -> OR10/1
  HvCoorn_pctHVBatSocEER/1 -> Switch17/1
  Switch17/1 -> HvCoorn_pctHVBatSocEEW/1, Equal5/1
  hpp_tiRemHvBatPrecdngSet_C32/1 -> Equal5/2
  idi_noBMSSocCounter/1 -> Equal7/1
  uint15/1 -> Equal7/2
  hpp_tiRemHvBatPrecdngSet_C33/1 -> TurnOnDelayVari6/3
  Equal7/1 -> TurnOnDelayVari6/1
  TaskTime_s13/1 -> TurnOnDelayVari6/2
  [iud_bEEIniFnsd] -> AND40/1
  AND40/1 -> Switch17/2
  [icbms_pctHVBatSOCDisp] -> Switch17/3
  Not9/1 -> AND40/2
  TurnOnDelayVari6/1 -> Not9/1
  Equal5/1 -> OR12/1
  OR12/1 -> AND37/2
  hpp_tiRemHvBatPrecdngSet_C34/1 -> OR12/2
  Not8/1 -> OR13/1
  OR13/1 -> AND23/2

== system HvCoorn/HvCoorn/HVP_HighVoltagePowerOnOffProcedure/A01_HighvoltPowerUpReq/B15_LbmsMntn ==
  iclbms_stLvRemChrgReq : Inport
  icbms_pctHVBatSOCDisp : Inport  Port=2
  HvCoorn_stHVPOld : Inport  Port=3
  icdc_stMode : Inport  Port=4
  HvCoorn_ctSmtBatMntnFailEER : Inport  Port=5
  iud_bEEIniFnsd : Inport  Port=6
  ipf_bLBMSCANVld : Inport  Port=7
  idi_bKeyOn : Inport  Port=8
  AND{,1..2,19} (4 alike) : Logic  OutDataTypeStr=boolean
  Add : Sum  InputSameDT=on  SaturateOnIntegerOverflow=on
  Add1 : Sum  InputSameDT=on  SaturateOnIntegerOverflow=on
  EdgeRising1 : ITKLib/Memory/EdgeRising  Tag=initial value = 0
      settings: SourceProductName=ITKC_Lib
  EdgeRising2 : ITKLib/Memory/EdgeRising  Tag=initial value = 0
      settings: SourceProductName=ITKC_Lib
  EdgeRising3 : ITKLib/Memory/EdgeRising  Tag=initial value = 0
      settings: SourceProductName=ITKC_Lib
  Equal{1..4} (4 alike) : RelationalOperator  Operator===  OutDataTypeStr=boolean
  Greater1 : RelationalOperator  OutDataTypeStr=boolean
  Greater15 : RelationalOperator  Operator=~=  OutDataTypeStr=boolean
  Greater16 : RelationalOperator  Operator=~=  OutDataTypeStr=boolean
  Greater2 : RelationalOperator  Operator=<  OutDataTypeStr=boolean
  Not : Logic  Operator=NOT  AllPortsSameDT=off  OutDataTypeStr=boolean
  Not1 : Logic  Operator=NOT  AllPortsSameDT=off  OutDataTypeStr=boolean
  OR1 : Logic  Operator=OR  OutDataTypeStr=boolean
  OR2 : Logic  Operator=OR  OutDataTypeStr=boolean
  OR3 : Logic  Operator=OR  OutDataTypeStr=boolean
  OR4 : Logic  Operator=OR  Inputs=3  OutDataTypeStr=boolean
  RSLatch : ITKLib/Memory/RSLatch
      settings: SourceProductName=ITKC_Lib
  RSLatch1 : ITKLib/Memory/RSLatch
      settings: SourceProductName=ITKC_Lib
  Relational Operator1 : RelationalOperator  Operator===  OutDataTypeStr=boolean  InputSameDT=off
  Relational Operator5 : RelationalOperator  Operator=~=  OutDataTypeStr=boolean  InputSameDT=off
  Switch : Switch  Criteria=u2 ~= 0  SaturateOnIntegerOverflow=off  InputSameDT=off
      settings: AttributesFormatString=Criteria : %<Criteria>
  Switch1 : Switch  Criteria=u2 ~= 0  SaturateOnIntegerOverflow=off  InputSameDT=off
      settings: AttributesFormatString=Criteria : %<Criteria>
  Switch2 : Switch  Criteria=u2 ~= 0  SaturateOnIntegerOverflow=off  InputSameDT=off
      settings: AttributesFormatString=Criteria : %<Criteria>
  TaskTime_s1 : Constant  Value=TaskTime_10ms
      settings: AttributesFormatString=[0.01]
  TaskTime_s3 : Constant  Value=TaskTime_10ms
      settings: AttributesFormatString=[0.01]
  TaskTime_s4 : Constant  Value=TaskTime_10ms
      settings: AttributesFormatString=[0.01]
  TurnOnDelayVari : ITKLib/TimeCounter/TurnOnDelayVari
      settings: AttributesFormatString=TurnOnDelay  SourceProductName=ITKC_Lib
  TurnOnDelayVari3 : ITKLib/TimeCounter/TurnOnDelayVari
      settings: AttributesFormatString=TurnOnDelay  SourceProductName=ITKC_Lib
  TurnOnDelayVari4 : ITKLib/TimeCounter/TurnOnDelayVari
      settings: AttributesFormatString=TurnOnDelay  SourceProductName=ITKC_Lib
  Unit Delay : UnitDelay  SampleTime=-1  HasFrameUpgradeWarning=on
      settings: AttributesFormatString=<initial=%<x0>>
  UnitDelay : UnitDelay  SampleTime=-1  HasFrameUpgradeWarning=on
      settings: AttributesFormatString=<Initial=%<x0>>
  hpp_tiRemHvBatPrecdngSet_C1 : Constant  Description=[3600]  Value=HvCoorn_tiMntnLbmsInvldThd_C
      settings: AttributesFormatString=%<Description>
  hpp_tiRemHvBatPrecdngSet_C2 : Constant  Description=[50]  Value=HvCoorn_pctLbmsSocMntnThd_C
      settings: AttributesFormatString=%<Description>
  hpp_tiRemHvBatPrecdngSet_C6 : Constant  Description=[10]  Value=HvCoorn_pctHvSocLbmsMntnDisb_C
      settings: AttributesFormatString=%<Description>
  hpp_tiRemHvBatPrecdngSet_C7 : Constant  Description=[3]  Value=HvCoorn_ctFailLbmsMntnDisb_C
      settings: AttributesFormatString=%<Description>
  hpp_tiRemHvBatPrecdngSet_C8 : Constant  Description=[15]  Value=HvCoorn_tiMntnFailNoRdyThd_C
      settings: AttributesFormatString=%<Description>
  hpp_tiRemHvBatPrecdngSet_C9 : Constant  Description=[15]  Value=HvCoorn_tiMntnFailNoBuckThd_C
      settings: AttributesFormatString=%<Description>
  icdc_disconnected : Constant  Description=[1]  Value=DCDCActSt_buck
      settings: AttributesFormatString=[1]
  icdc_disconnected1 : Constant  Description=[1]  Value=DCDCActSt_buck
      settings: AttributesFormatString=[1]
  uint1 : Constant  OutDataTypeStr=uint8  SampleTime=-1
      settings: AttributesFormatString=%<OutDataTypeStr>
  uint2 : Constant  Value=4  OutDataTypeStr=uint8  SampleTime=-1
      settings: AttributesFormatString=%<OutDataTypeStr>
  uint3 : Constant  Value=0  OutDataTypeStr=uint8  SampleTime=-1
      settings: AttributesFormatString=%<OutDataTypeStr>
  uint4 : Constant  Value=0  OutDataTypeStr=uint8  SampleTime=-1
      settings: AttributesFormatString=%<OutDataTypeStr>
  uint5 : Constant  OutDataTypeStr=uint8  SampleTime=-1
      settings: AttributesFormatString=%<OutDataTypeStr>
  uint6 : Constant  Value=89  OutDataTypeStr=uint8  SampleTime=-1
      settings: AttributesFormatString=%<OutDataTypeStr>
  uint7 : Constant  Value=90  OutDataTypeStr=uint8  SampleTime=-1
      settings: AttributesFormatString=%<OutDataTypeStr>
  uint8 : Constant  OutDataTypeStr=uint8  SampleTime=-1
      settings: AttributesFormatString=%<OutDataTypeStr>
  HvCoorn_ctLbmsMntnFailEEW : Outport  VectorParamsAs1DForOutWhenUnconnected=off
  HvCoorn_bLbmsLvBatMntnReq : Outport  Port=2  VectorParamsAs1DForOutWhenUnconnected=off
  HvCoorn_pctLbmsSocMntnThd : Outport  Port=3  VectorParamsAs1DForOutWhenUnconnected=off
  HvCoorn_bLbmsSocWkup : Outport  Port=4  VectorParamsAs1DForOutWhenUnconnected=off
  wires:
  iclbms_stLvRemChrgReq/1 -> [iclbms_stLvRemChrgReq], Equal1/1, Equal4/1, Equal3/1
  uint8/1 -> Equal1/2  "SOCChar"
  hpp_tiRemHvBatPrecdngSet_C2/1 -> HvCoorn_pctLbmsSocMntnThd/1
  RSLatch/1 -> UnitDelay/1, HvCoorn_bLbmsLvBatMntnReq/1
  UnitDelay/1 -> [HvCoorn_bLbmsMntnReqOld]
  icbms_pctHVBatSOCDisp/1 -> Greater2/1
  hpp_tiRemHvBatPrecdngSet_C6/1 -> Greater2/2
  Greater2/1 -> OR1/1
  Greater1/1 -> OR1/2
  [HvCoorn_ctLbmsMntnFailEEW] -> Greater1/1
  hpp_tiRemHvBatPrecdngSet_C7/1 -> Greater1/2
  OR1/1 -> Not/1
  Not/1 -> HvCoorn_bLbmsSocWkup/1
  uint1/1 -> Equal2/2  "SOCChar"
  [iclbms_stLvRemChrgReq] -> Equal2/1
  uint7/1 -> Greater16/2
  Greater15/1 -> AND19/1
  HvCoorn_stHVPOld/1 -> Greater16/1, Greater15/1
  uint6/1 -> Greater15/2
  Greater16/1 -> AND19/2
  Equal2/1 -> AND1/2
  AND19/1 -> AND1/1
  hpp_tiRemHvBatPrecdngSet_C8/1 -> TurnOnDelayVari3/3
  TaskTime_s3/1 -> TurnOnDelayVari3/2
  AND1/1 -> TurnOnDelayVari3/1
  icdc_disconnected/1 -> Relational Operator5/2
  icdc_stMode/1 -> [icdc_stMode], Relational Operator5/1
  Relational Operator5/1 -> AND2/2
  TaskTime_s4/1 -> TurnOnDelayVari4/2
  hpp_tiRemHvBatPrecdngSet_C9/1 -> TurnOnDelayVari4/3
  AND2/1 -> TurnOnDelayVari4/1
  OR2/1 -> EdgeRising2/1
  EdgeRising1/1 -> Switch/2
  Add/1 -> Switch/1
  HvCoorn_ctSmtBatMntnFailEER/1 -> Add/1
  Switch/1 -> Switch2/3
  Switch1/1 -> Add/2, Switch/3
  uint5/1 -> Add1/2
  iud_bEEIniFnsd/1 -> EdgeRising1/1
  Add1/1 -> Switch1/1
  Unit Delay/1 -> Add1/1, Switch1/3
  uint4/1 -> Switch2/1
  Switch2/1 -> [HvCoorn_ctLbmsMntnFailEEW], Unit Delay/1, HvCoorn_ctLbmsMntnFailEEW/1
  Equal1/1 -> RSLatch/1
  uint2/1 -> Equal3/2  "CharQuit"
  ipf_bLBMSCANVld/1 -> Not1/1
  [HvCoorn_bLbmsMntnReqOld] -> TurnOnDelayVari/1
  TaskTime_s1/1 -> TurnOnDelayVari/2
  hpp_tiRemHvBatPrecdngSet_C1/1 -> TurnOnDelayVari/3
  TurnOnDelayVari/1 -> AND/2
  Not1/1 -> AND/1
  OR3/1 -> RSLatch1/2, OR4/1
  OR4/1 -> RSLatch/2
  [HvCoorn_bLbmsMntnReqOld] -> AND2/1
  icdc_disconnected1/1 -> Relational Operator1/2
  [icdc_stMode] -> Relational Operator1/1
  Relational Operator1/1 -> EdgeRising3/1
  EdgeRising3/1 -> Switch2/2
  AND/1 -> RSLatch1/1
  RSLatch1/1 -> OR4/2
  TurnOnDelayVari3/1 -> OR2/1
  TurnOnDelayVari4/1 -> OR2/2
  EdgeRising2/1 -> Switch1/2
  uint3/1 -> Equal4/2
  Equal3/1 -> OR3/1
  Equal4/1 -> OR3/2
  idi_bKeyOn/1 -> OR4/3

== system HvCoorn/HvCoorn/HVP_HighVoltagePowerOnOffProcedure/A01_HighvoltPowerUpReq/B16_LvBattTypSwt ==
  VehCfg_stLvBattTyp : Inport
  HvCoorn_ctSmtBatMntnFailEEW1 : Inport  Port=2
  HvCoorn_bLvBatMntnReq : Inport  Port=3
  HvCoorn_ctLbmsMntnFailEEW : Inport  Port=4
  HvCoorn_bLbmsLvBatMntnReq : Inport  Port=5
  Constant84 : Constant  Description=[1]  Value=LvBattTyp_stLiBatt_SC
      settings: AttributesFormatString=%<Description>
  Equal3 : RelationalOperator  Operator===  OutDataTypeStr=boolean
  Switch : Switch  Criteria=u2 ~= 0  SaturateOnIntegerOverflow=off  InputSameDT=off
      settings: AttributesFormatString=Criteria : %<Criteria>
  Switch1 : Switch  Criteria=u2 ~= 0  SaturateOnIntegerOverflow=off  InputSameDT=off
      settings: AttributesFormatString=Criteria : %<Criteria>
  HvCoorn_ctSmtBatMntnFailEEW : Outport
  HvCoorn_bRemLvBatMntnReq : Outport  Port=2
  wires:
  Constant84/1 -> Equal3/2
  Equal3/1 -> Switch1/2, Switch/2
  Switch/1 -> HvCoorn_ctSmtBatMntnFailEEW/1
  VehCfg_stLvBattTyp/1 -> Equal3/1
  HvCoorn_ctSmtBatMntnFailEEW1/1 -> Switch/3
  HvCoorn_ctLbmsMntnFailEEW/1 -> Switch/1
  HvCoorn_bLvBatMntnReq/1 -> Switch1/3
  HvCoorn_bLbmsLvBatMntnReq/1 -> Switch1/1
  Switch1/1 -> HvCoorn_bRemLvBatMntnReq/1

== system HvCoorn/HvCoorn/HVP_HighVoltagePowerOnOffProcedure/A30_Authcation/B01_Warnning ==
  note: 0x0:No warning0x1:Warning Level 1(3-5)
      | 0x2:Warning Level 2(6-10)
      | 0x3:Warning Level 3(11-14)
  HvCoorn_authfailed_conter : Inport
  idi_bKeyOn : Inport  Port=2
  AND1 : Logic  OutDataTypeStr=boolean
  EdgeRising2 : ITKLib/Memory/EdgeRising  Tag=initial value = 0
      settings: SourceProductName=ITKC_Lib
  Equal : RelationalOperator  Operator===  OutDataTypeStr=boolean  RndMeth=Simplest  InputSameDT=off
  Equal1 : RelationalOperator  OutDataTypeStr=boolean  RndMeth=Simplest  InputSameDT=off
  Equal2 : RelationalOperator  OutDataTypeStr=boolean  RndMeth=Simplest  InputSameDT=off
  Equal9 : RelationalOperator  OutDataTypeStr=boolean  RndMeth=Simplest  InputSameDT=off
  Not1 : Logic  Operator=NOT  AllPortsSameDT=off  OutDataTypeStr=boolean
  RSLatch : ITKLib/Memory/RSLatch
      settings: SourceProductName=ITKC_Lib
  Switch{,1..2,9..10} (5 alike) : Switch  Criteria=u2 ~= 0  SaturateOnIntegerOverflow=off  InputSameDT=off
      settings: AttributesFormatString=Criteria : %<Criteria>
  TaskTime_s2 : Constant  Value=TaskTime_10ms
      settings: AttributesFormatString=[0.01]
  Turn_Off_Delay_Vari1 : ITKLib/TimeCounter/Turn_Off_Delay_Vari
      settings: AttributesFormatString=TurnOffDelay  SourceProductName=ITKC_Lib
  sup_tiChgConndown_C : Constant  Description=[0.03]  Value=HvCoorn_tiSpeed20LimitDly_C
      settings: AttributesFormatString=%<Description>
  sup_tiChgConndown_C1 : Constant  Description=[0]  Value=HvCoorn_bAuthFailSpdLimOvrd_C
      settings: AttributesFormatString=%<Description>
  sup_tiChgConndown_C2 : Constant  Description=[0]  Value=HvCoorn_bAuthFailSpdLimOvrdVal_C
      settings: AttributesFormatString=%<Description>
  sup_tiChgConndown_C3 : Constant  Description=[0]  Value=HvCoorn_stAuthChkFailLvlOvrd_C
      settings: AttributesFormatString=%<Description>
  sup_tiChgConndown_C4 : Constant  Description=[0]  Value=HvCoorn_stAuthChkFailLvlOvrdVal_C
      settings: AttributesFormatString=%<Description>
  uint1 : Constant  Value=3  OutDataTypeStr=uint8  SampleTime=-1
      settings: AttributesFormatString=%<OutDataTypeStr>
  uint10 : Constant  Value=15  OutDataTypeStr=uint8  SampleTime=-1
      settings: AttributesFormatString=%<OutDataTypeStr>
  uint17 : Constant  Value=11  OutDataTypeStr=uint8  SampleTime=-1
      settings: AttributesFormatString=%<OutDataTypeStr>
  uint2 : Constant  OutDataTypeStr=uint8  SampleTime=-1
      settings: AttributesFormatString=%<OutDataTypeStr>
  uint4 : Constant  Value=2  OutDataTypeStr=uint8  SampleTime=-1
      settings: AttributesFormatString=%<OutDataTypeStr>
  uint7 : Constant  Value=0  OutDataTypeStr=uint8  SampleTime=-1
      settings: AttributesFormatString=%<OutDataTypeStr>
  uint8 : Constant  Value=6  OutDataTypeStr=uint8  SampleTime=-1
      settings: AttributesFormatString=%<OutDataTypeStr>
  uint9 : Constant  Value=3  OutDataTypeStr=uint8  SampleTime=-1
      settings: AttributesFormatString=%<OutDataTypeStr>
  HvCoorn_stAuthChkFailLvl : Outport
  HvCoorn_bAuthFailSpdLim : Outport  Port=2  VectorParamsAs1DForOutWhenUnconnected=off
  wires:
  uint1/1 -> Equal1/2
  uint7/1 -> Switch9/3
  Switch10/1 -> Switch/3
  uint2/1 -> Switch9/1
  Equal1/1 -> Switch9/2
  Equal2/1 -> Switch10/2
  Switch9/1 -> Switch10/3
  uint8/1 -> Equal2/2
  uint4/1 -> Switch10/1
  uint9/1 -> Switch/1
  Equal9/1 -> Switch/2
  uint17/1 -> Equal9/2
  Switch/1 -> Switch1/3
  uint10/1 -> Equal/2
  HvCoorn_authfailed_conter/1 -> Equal1/1, Equal2/1, Equal9/1, [HvCoorn_authfailed_conter]
  EdgeRising2/1 -> AND1/1
  Turn_Off_Delay_Vari1/1 -> Not1/1
  Equal/1 -> AND1/2
  AND1/1 -> RSLatch/1
  [HvCoorn_authfailed_conter] -> Equal/1
  sup_tiChgConndown_C/1 -> Turn_Off_Delay_Vari1/3
  idi_bKeyOn/1 -> Turn_Off_Delay_Vari1/1, EdgeRising2/1
  TaskTime_s2/1 -> Turn_Off_Delay_Vari1/2
  Not1/1 -> RSLatch/2
  Switch1/1 -> HvCoorn_stAuthChkFailLvl/1
  Switch2/1 -> HvCoorn_bAuthFailSpdLim/1
  RSLatch/1 -> Switch2/3
  sup_tiChgConndown_C1/1 -> Switch2/2
  sup_tiChgConndown_C2/1 -> Switch2/1
  sup_tiChgConndown_C3/1 -> Switch1/2
  sup_tiChgConndown_C4/1 -> Switch1/1

== system HvCoorn/HvCoorn/HVP_HighVoltagePowerOnOffProcedure/A30_Authcation/Subsystem ==
  HvCoorn_stTboxByte7Req : Inport
  Add3 : Sum  Inputs=++++  SaturateOnIntegerOverflow=on
  Add4 : Sum  Inputs=++++  SaturateOnIntegerOverflow=on
  Constant1 : Constant  Value=7
  Constant11 : Constant
  Constant12 : Constant  Value=2
  Constant13 : Constant  Value=3
  Constant14 : Constant  Value=4
  Constant15 : Constant  Value=5
  Constant16 : Constant  Value=6
  Constant2 : Constant  Value=0
  Data Type Conversion{,1..9} (10 alike) : DataTypeConversion  SaturateOnIntegerOverflow=off  RndMeth=Floor
  Gain10 : Gain  Gain=4  OutDataTypeStr=uint8
  Gain11 : Gain  Gain=8  OutDataTypeStr=uint8
  Gain12 : Gain  OutDataTypeStr=uint8
  Gain13 : Gain  Gain=2  OutDataTypeStr=uint8
  Gain14 : Gain  Gain=4  OutDataTypeStr=uint8
  Gain15 : Gain  Gain=8  OutDataTypeStr=uint8
  Gain8 : Gain  OutDataTypeStr=uint8
  Gain9 : Gain  Gain=2  OutDataTypeStr=uint8
  Saturation : Saturate  UpperLimit=15  LowerLimit=0  OutDataTypeStr=uint8
  Saturation1 : Saturate  UpperLimit=15  LowerLimit=0  OutDataTypeStr=uint8
  Subsystem{9..16} (8 alike) : ITKLib/BitOperation/Subsystem1
      settings: SourceProductName=ITKC_Lib
  TBOX_Instruction_Type_req : Outport  VectorParamsAs1DForOutWhenUnconnected=off
  TBOX_receiver_module_req : Outport  Port=2  VectorParamsAs1DForOutWhenUnconnected=off
  wires:
  Saturation/1 -> TBOX_receiver_module_req/1  "TBOX_receiver_module_req"
  Saturation1/1 -> TBOX_Instruction_Type_req/1  "TBOX_Instruction_Type_req"
  Data Type Conversion/1 -> Saturation/1
  Data Type Conversion1/1 -> Saturation1/1
  Data Type Conversion5/1 -> Gain15/1
  Subsystem13/1 -> Data Type Conversion6/1
  Data Type Conversion8/1 -> Gain10/1
  Data Type Conversion4/1 -> Gain14/1
  Data Type Conversion7/1 -> Gain9/1
  Data Type Conversion6/1 -> Gain8/1
  Subsystem15/1 -> Data Type Conversion8/1
  Subsystem14/1 -> Data Type Conversion7/1
  Data Type Conversion2/1 -> Gain12/1
  Subsystem16/1 -> Data Type Conversion9/1
  Add3/1 -> Data Type Conversion1/1
  Constant12/1 -> Subsystem11/1
  Gain13/1 -> Add4/2
  Subsystem10/1 -> Data Type Conversion3/1
  Gain11/1 -> Add3/4
  Gain9/1 -> Add3/2
  Data Type Conversion3/1 -> Gain13/1
  Constant2/1 -> Subsystem9/1
  Gain8/1 -> Add3/1
  Constant11/1 -> Subsystem10/1
  Constant14/1 -> Subsystem13/1
  Data Type Conversion9/1 -> Gain11/1
  Constant15/1 -> Subsystem14/1
  Gain15/1 -> Add4/4
  Add4/1 -> Data Type Conversion/1
  Subsystem9/1 -> Data Type Conversion2/1
  Subsystem12/1 -> Data Type Conversion5/1
  Constant1/1 -> Subsystem16/1
  Constant13/1 -> Subsystem12/1
  HvCoorn_stTboxByte7Req/1 -> Subsystem9/2, Subsystem10/2, Subsystem11/2, Subsystem13/2, Subsystem16/2, Subsystem15/2, Subsystem14/2, Subsystem12/2
  Gain14/1 -> Add4/3
  Gain10/1 -> Add3/3
  Subsystem11/1 -> Data Type Conversion4/1
  Constant16/1 -> Subsystem15/1
  Gain12/1 -> Add4/1
